simulink model "project2_sim"  (R2022b)
settings: Solver=VariableStepAuto  StartTime=0.0  StopTime=10.0  RelTol=1e-3
values from neighbouring files (symbols this model uses):
  A = [ ... (first row only)    [project2.m]    (also in project2_p1.m = A-B*K_reg; project2_p2.m = A-B*K_reg)
  Ad = [ ... (first row only)    [project2.m]    (also in project2_p2.m; set_topology.m)
  B = [ ... (first row only)    [project2.m]    (also in project2_p1.m; project2_p2.m)
  c = (0.5/min(real(eigs)))+ 0.5    [project2_p1.m]    (also in project2_p2.m = (0.5/min(real(eigs))) + 0.5)
  C = [708.27 0]    [project2.m]    (also in project2_p1.m; project2_p2.m)
  F = Pf*C'/R    [project2_p1.m]
  G = [ ... (first row only)    [project2.m]    (also in project2_p2.m = eye(6); set_topology.m = diag([1 0 0 0 0 1]))
  K = R\B'*P    [project2_p1.m]    (also in project2_p2.m = inv(R)*B'*P)
  K_reg = acker(A,B, [0 0])    [project2_p1.m]    (also in project2_p2.m)
  Lu_obs = (place(A', C', [-20, -10]))'    [project2_p1.m]
  xhat0 = [0 0]'    [project2_p1.m]    (also in project2_p2.m)
settings Model: Creator=simonecarena  LastModifiedBy=Enf
settings DebuggingCC: AlgebraicLoopMsg=none

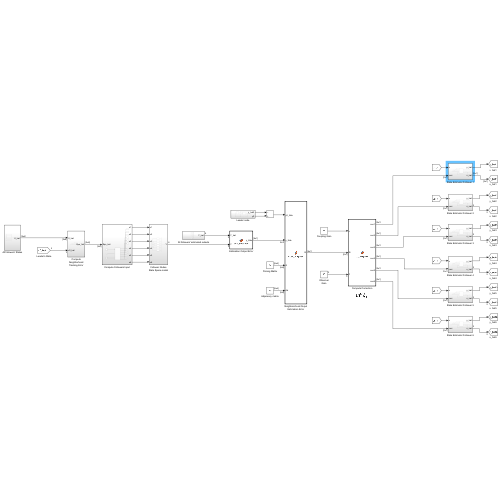
[thumbnail: Simulink's stored preview of the top-level diagram]
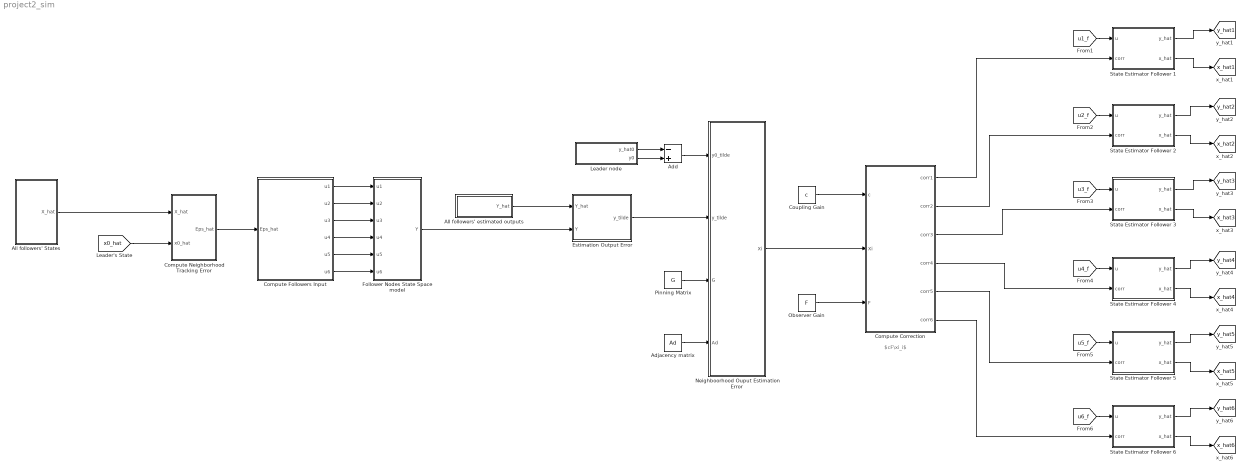
== system project2_sim ==
  note: $cF\xi_i$
  Add : Sum  Inputs=-+
  Adjacency matrix : Constant  Value=Ad
  All followers' States : Subsystem
  All followers' estimated outputs : Subsystem
  Compute Neighborhood Tracking Error : Subsystem
  Compute Correction : MATLAB Function  TreatAsAtomicUnit=on
  Compute Followers Input : Subsystem
  Coupling Gain : Constant  Value=c
  Estimation Output Error : MATLAB Function  TreatAsAtomicUnit=on
  Follower Nodes State Space model : Subsystem
  Leader node : Subsystem
  Neighboorhood Ouput Estimation Error : MATLAB Function  TreatAsAtomicUnit=on
  Observer Gain : Constant  Value=F
  Pinning Matrix : Constant  Value=G
  State Estimator Follower 1 : Subsystem
  State Estimator Follower 2 : Subsystem
  State Estimator Follower 3 : Subsystem
  State Estimator Follower 4 : Subsystem
  State Estimator Follower 5 : Subsystem
  State Estimator Follower 6 : Subsystem
  tag scope: x_hat1=global, x_hat2=global, x_hat3=global, x_hat4=global, x_hat5=global, x_hat6=global, y_hat1=global, y_hat2=global, y_hat3=global, y_hat4=global, y_hat5=global, y_hat6=global
  wires:
  Estimation Output Error/1(y_tilde) -> Neighboorhood Ouput Estimation Error/2(y_tilde)
  Adjacency matrix/1 -> Neighboorhood Ouput Estimation Error/4(Ad)
  Pinning Matrix/1 -> Neighboorhood Ouput Estimation Error/3(G)
  Add/1 -> Neighboorhood Ouput Estimation Error/1(y0_tilde)
  Neighboorhood Ouput Estimation Error/1(Xi) -> Compute Correction/2(Xi)
  Compute Correction/1(corr1) -> State Estimator Follower 1/2(corr)
  Compute Correction/2(corr2) -> State Estimator Follower 2/2(corr)
  Compute Correction/3(corr3) -> State Estimator Follower 3/2(corr)
  Compute Correction/4(corr4) -> State Estimator Follower 4/2(corr)
  Compute Correction/5(corr5) -> State Estimator Follower 5/2(corr)
  Compute Correction/6(corr6) -> State Estimator Follower 6/2(corr)
  State Estimator Follower 1/1(y_hat) -> [y_hat1]
  State Estimator Follower 3/1(y_hat) -> [y_hat3]
  State Estimator Follower 6/1(y_hat) -> [y_hat6]
  State Estimator Follower 5/1(y_hat) -> [y_hat5]
  State Estimator Follower 4/1(y_hat) -> [y_hat4]
  State Estimator Follower 2/1(y_hat) -> [y_hat2]
  All followers' estimated outputs/1(Y_hat) -> Estimation Output Error/1(Y_hat)
  State Estimator Follower 1/2(x_hat) -> [x_hat1]
  State Estimator Follower 2/2(x_hat) -> [x_hat2]
  State Estimator Follower 3/2(x_hat) -> [x_hat3]
  State Estimator Follower 4/2(x_hat) -> [x_hat4]
  State Estimator Follower 5/2(x_hat) -> [x_hat5]
  State Estimator Follower 6/2(x_hat) -> [x_hat6]
  Leader node/1(y_hat0) -> Add/1
  Leader node/2(y0) -> Add/2
  Observer Gain/1 -> Compute Correction/3(F)
  Coupling Gain/1 -> Compute Correction/1(c)
  All followers' States/1(X_hat) -> Compute Neighborhood Tracking Error/1(X_hat)
  [x0_hat] -> Compute Neighborhood Tracking Error/2(x0_hat)
  Compute Neighborhood Tracking Error/1(Eps_hat) -> Compute Followers Input/1(Eps_hat)
  [u4_f] -> State Estimator Follower 4/1(u)
  [u6_f] -> State Estimator Follower 6/1(u)
  [u5_f] -> State Estimator Follower 5/1(u)
  [u3_f] -> State Estimator Follower 3/1(u)
  [u1_f] -> State Estimator Follower 1/1(u)
  [u2_f] -> State Estimator Follower 2/1(u)
  Compute Followers Input/1(u1) -> Follower Nodes State Space model/1(u1)
  Compute Followers Input/2(u2) -> Follower Nodes State Space model/2(u2)
  Compute Followers Input/3(u3) -> Follower Nodes State Space model/3(u3)
  Compute Followers Input/4(u4) -> Follower Nodes State Space model/4(u4)
  Compute Followers Input/5(u5) -> Follower Nodes State Space model/5(u5)
  Compute Followers Input/6(u6) -> Follower Nodes State Space model/6(u6)
  Follower Nodes State Space model/1(Y) -> Estimation Output Error/2(Y)

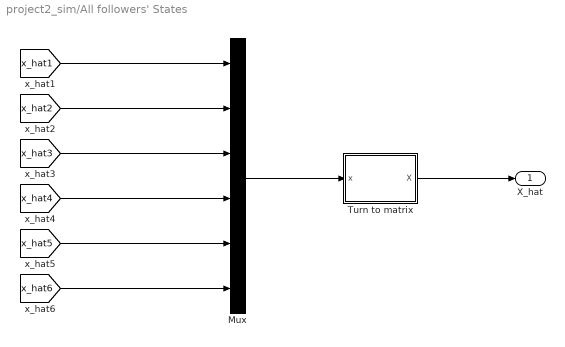
== system project2_sim/All followers' States ==
  Mux : Mux  Inputs=6
  Turn to matrix : MATLAB Function  TreatAsAtomicUnit=on
  X_hat : Outport
  wires:
  [x_hat1] -> Mux/1
  [x_hat2] -> Mux/2
  [x_hat3] -> Mux/3
  [x_hat4] -> Mux/4
  [x_hat5] -> Mux/5
  [x_hat6] -> Mux/6
  Mux/1 -> Turn to matrix/1(x)
  Turn to matrix/1(X) -> X_hat/1

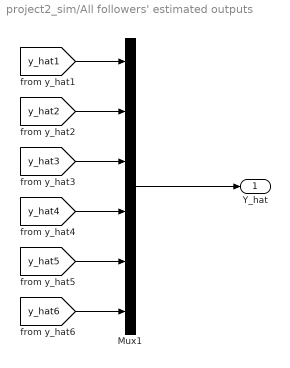
== system project2_sim/All followers' estimated outputs ==
  Mux1 : Mux  Inputs=6
  Y_hat : Outport
  wires:
  [y_hat6] -> Mux1/6
  [y_hat4] -> Mux1/4
  [y_hat1] -> Mux1/1
  [y_hat5] -> Mux1/5
  [y_hat3] -> Mux1/3
  Mux1/1 -> Y_hat/1
  [y_hat2] -> Mux1/2

== system project2_sim/Compute Neighborhood Tracking Error ==
  X_hat : Inport
  x0_hat : Inport  Port=2
  Constant1 : Constant  Value=G
  Neighborhood Tracking Error : MATLAB Function  TreatAsAtomicUnit=on
  adjacency matrix : Constant  Value=Ad
  Eps_hat : Outport
  wires:
  X_hat/1 -> Neighborhood Tracking Error/1(X_hat)
  x0_hat/1 -> Neighborhood Tracking Error/2(x0_hat)
  adjacency matrix/1 -> Neighborhood Tracking Error/3(Ad)
  Constant1/1 -> Neighborhood Tracking Error/4(G)
  Neighborhood Tracking Error/1(Eps) -> Eps_hat/1

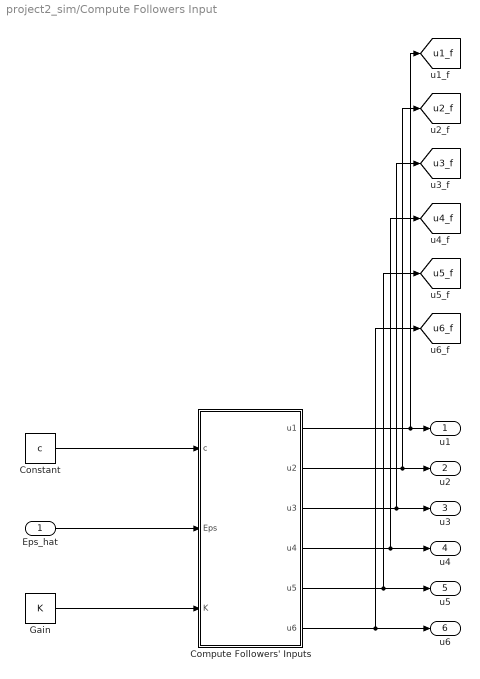
== system project2_sim/Compute Followers Input ==
  Eps_hat : Inport
  Compute Followers' Inputs : MATLAB Function  TreatAsAtomicUnit=on
  Constant : Constant  Value=c
  Gain : Constant  Value=K  VectorParams1D=off
  u1 : Outport
  u2 : Outport  Port=2
  u3 : Outport  Port=3
  u4 : Outport  Port=4
  u5 : Outport  Port=5
  u6 : Outport  Port=6
  tag scope: u1_f=global, u2_f=global, u3_f=global, u4_f=global, u5_f=global, u6_f=global
  wires:
  Eps_hat/1 -> Compute Followers' Inputs/2(Eps)
  Constant/1 -> Compute Followers' Inputs/1(c)
  Gain/1 -> Compute Followers' Inputs/3(K)
  Compute Followers' Inputs/1(u1) -> [u1_f], u1/1
  Compute Followers' Inputs/2(u2) -> u2/1, [u2_f]
  Compute Followers' Inputs/3(u3) -> u3/1, [u3_f]
  Compute Followers' Inputs/4(u4) -> u4/1, [u4_f]
  Compute Followers' Inputs/5(u5) -> u5/1, [u5_f]
  Compute Followers' Inputs/6(u6) -> [u6_f], u6/1

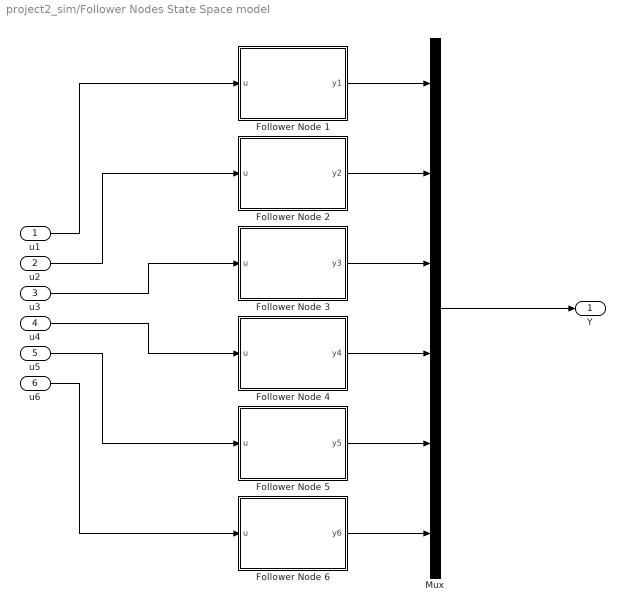
== system project2_sim/Follower Nodes State Space model ==
  u1 : Inport
  u2 : Inport  Port=2
  u3 : Inport  Port=3
  u4 : Inport  Port=4
  u5 : Inport  Port=5
  u6 : Inport  Port=6
  Follower Node 1 : Subsystem
  Follower Node 2 : Subsystem
  Follower Node 3 : Subsystem
  Follower Node 4 : Subsystem
  Follower Node 5 : Subsystem
  Follower Node 6 : Subsystem
  Mux : Mux  Inputs=6
  Y : Outport
  wires:
  Follower Node 4/1(y4) -> Mux/4
  Mux/1 -> Y/1
  u4/1 -> Follower Node 4/1(u)
  Follower Node 2/1(y2) -> Mux/2
  Follower Node 6/1(y6) -> Mux/6
  Follower Node 3/1(y3) -> Mux/3
  Follower Node 1/1(y1) -> Mux/1
  Follower Node 5/1(y5) -> Mux/5
  u5/1 -> Follower Node 5/1(u)
  u3/1 -> Follower Node 3/1(u)
  u2/1 -> Follower Node 2/1(u)
  u1/1 -> Follower Node 1/1(u)
  u6/1 -> Follower Node 6/1(u)

== system project2_sim/Leader node ==
  Gain : Gain  Gain=-K_reg  Multiplication=Matrix(K*u)
  Leader Node : Subsystem
  Leader Node Estimator : Subsystem
  y_hat0 : Outport
  y0 : Outport  Port=2
  wires:
  Leader Node Estimator/2(y_hat0) -> y_hat0/1
  Leader Node/1(y0) -> y0/1, Leader Node Estimator/1(y0)
  Gain/1 -> Leader Node/1(u), Leader Node Estimator/2(u)
  Leader Node Estimator/1(x_hat0) -> Gain/1

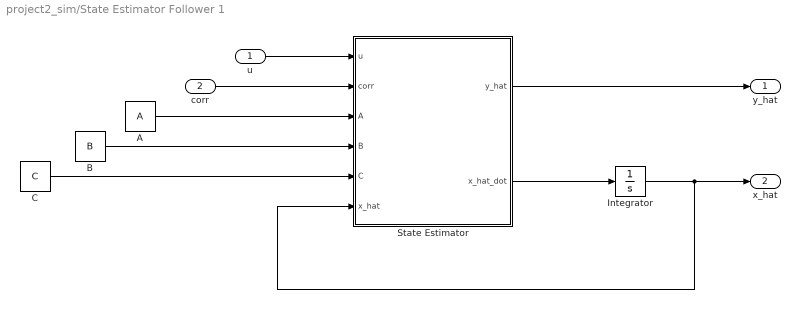
== system project2_sim/State Estimator Follower 1 ==
  u : Inport
  corr : Inport  Port=2
  A : Constant  Value=A
  B : Constant  Value=B  VectorParams1D=off
  C : Constant  Value=C  VectorParams1D=off
  Integrator : Integrator  InitialCondition=xhat0
  State Estimator : MATLAB Function  TreatAsAtomicUnit=on
  y_hat : Outport
  x_hat : Outport  Port=2
  wires:
  State Estimator/1(y_hat) -> y_hat/1
  u/1 -> State Estimator/1(u)
  corr/1 -> State Estimator/2(corr)
  State Estimator/2(x_hat_dot) -> Integrator/1
  Integrator/1 -> State Estimator/6(x_hat), x_hat/1
  A/1 -> State Estimator/3(A)
  B/1 -> State Estimator/4(B)
  C/1 -> State Estimator/5(C)

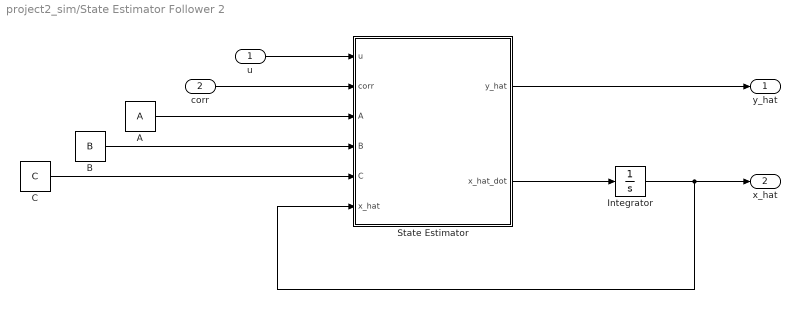
== system project2_sim/State Estimator Follower 2 ==
  u : Inport
  corr : Inport  Port=2
  A : Constant  Value=A
  B : Constant  Value=B  VectorParams1D=off
  C : Constant  Value=C  VectorParams1D=off
  Integrator : Integrator  InitialCondition=xhat0
  State Estimator : MATLAB Function  TreatAsAtomicUnit=on
  y_hat : Outport
  x_hat : Outport  Port=2
  wires:
  C/1 -> State Estimator/5(C)
  B/1 -> State Estimator/4(B)
  A/1 -> State Estimator/3(A)
  Integrator/1 -> x_hat/1, State Estimator/6(x_hat)
  State Estimator/2(x_hat_dot) -> Integrator/1
  corr/1 -> State Estimator/2(corr)
  u/1 -> State Estimator/1(u)
  State Estimator/1(y_hat) -> y_hat/1

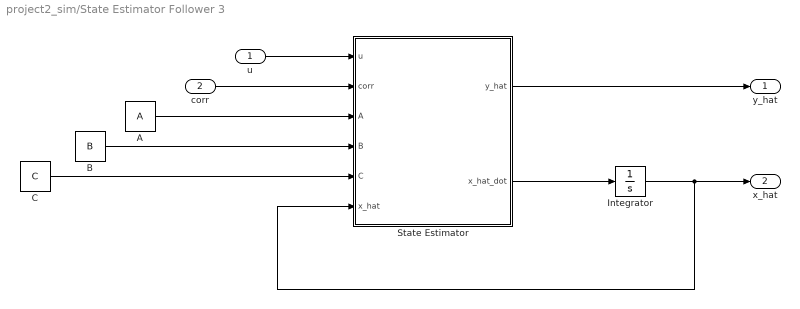
== system project2_sim/State Estimator Follower 3 ==
  u : Inport
  corr : Inport  Port=2
  A : Constant  Value=A
  B : Constant  Value=B  VectorParams1D=off
  C : Constant  Value=C  VectorParams1D=off
  Integrator : Integrator  InitialCondition=xhat0
  State Estimator : MATLAB Function  TreatAsAtomicUnit=on
  y_hat : Outport
  x_hat : Outport  Port=2
  wires:
  State Estimator/1(y_hat) -> y_hat/1
  u/1 -> State Estimator/1(u)
  corr/1 -> State Estimator/2(corr)
  State Estimator/2(x_hat_dot) -> Integrator/1
  Integrator/1 -> State Estimator/6(x_hat), x_hat/1
  A/1 -> State Estimator/3(A)
  B/1 -> State Estimator/4(B)
  C/1 -> State Estimator/5(C)

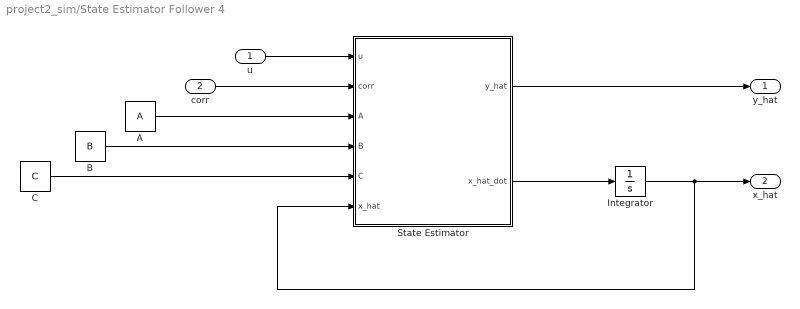
== system project2_sim/State Estimator Follower 4 ==
  u : Inport
  corr : Inport  Port=2
  A : Constant  Value=A
  B : Constant  Value=B  VectorParams1D=off
  C : Constant  Value=C  VectorParams1D=off
  Integrator : Integrator  InitialCondition=xhat0
  State Estimator : MATLAB Function  TreatAsAtomicUnit=on
  y_hat : Outport
  x_hat : Outport  Port=2
  wires:
  C/1 -> State Estimator/5(C)
  B/1 -> State Estimator/4(B)
  A/1 -> State Estimator/3(A)
  Integrator/1 -> x_hat/1, State Estimator/6(x_hat)
  State Estimator/2(x_hat_dot) -> Integrator/1
  corr/1 -> State Estimator/2(corr)
  u/1 -> State Estimator/1(u)
  State Estimator/1(y_hat) -> y_hat/1

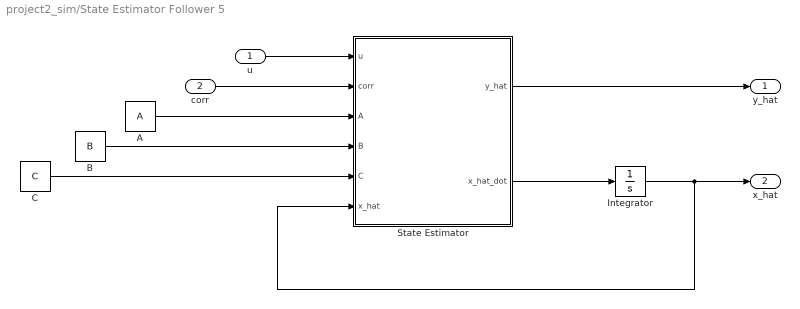
== system project2_sim/State Estimator Follower 5 ==
  u : Inport
  corr : Inport  Port=2
  A : Constant  Value=A
  B : Constant  Value=B  VectorParams1D=off
  C : Constant  Value=C  VectorParams1D=off
  Integrator : Integrator  InitialCondition=xhat0
  State Estimator : MATLAB Function  TreatAsAtomicUnit=on
  y_hat : Outport
  x_hat : Outport  Port=2
  wires:
  State Estimator/1(y_hat) -> y_hat/1
  u/1 -> State Estimator/1(u)
  corr/1 -> State Estimator/2(corr)
  State Estimator/2(x_hat_dot) -> Integrator/1
  Integrator/1 -> State Estimator/6(x_hat), x_hat/1
  A/1 -> State Estimator/3(A)
  B/1 -> State Estimator/4(B)
  C/1 -> State Estimator/5(C)

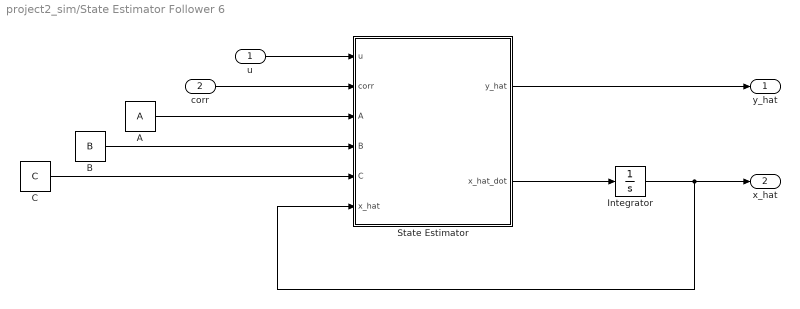
== system project2_sim/State Estimator Follower 6 ==
  u : Inport
  corr : Inport  Port=2
  A : Constant  Value=A
  B : Constant  Value=B  VectorParams1D=off
  C : Constant  Value=C  VectorParams1D=off
  Integrator : Integrator  InitialCondition=xhat0
  State Estimator : MATLAB Function  TreatAsAtomicUnit=on
  y_hat : Outport
  x_hat : Outport  Port=2
  wires:
  C/1 -> State Estimator/5(C)
  B/1 -> State Estimator/4(B)
  A/1 -> State Estimator/3(A)
  Integrator/1 -> x_hat/1, State Estimator/6(x_hat)
  State Estimator/2(x_hat_dot) -> Integrator/1
  corr/1 -> State Estimator/2(corr)
  u/1 -> State Estimator/1(u)
  State Estimator/1(y_hat) -> y_hat/1

== system project2_sim/Follower Nodes State Space model/Follower Node 1 ==
  u : Inport
  State-Space : StateSpace  A=A  B=B  C=C  D=0  InitialCondition=0
  y1 : Outport
  wires:
  u/1 -> State-Space/1
  State-Space/1 -> y1/1

== system project2_sim/Follower Nodes State Space model/Follower Node 2 ==
  u : Inport
  State-Space : StateSpace  A=A  B=B  C=C  D=0  InitialCondition=0
  y2 : Outport
  wires:
  u/1 -> State-Space/1
  State-Space/1 -> y2/1

== system project2_sim/Follower Nodes State Space model/Follower Node 3 ==
  u : Inport
  State-Space : StateSpace  A=A  B=B  C=C  D=0  InitialCondition=0
  y3 : Outport
  wires:
  u/1 -> State-Space/1
  State-Space/1 -> y3/1

== system project2_sim/Follower Nodes State Space model/Follower Node 4 ==
  u : Inport
  State-Space : StateSpace  A=A  B=B  C=C  D=0  InitialCondition=0
  y4 : Outport
  wires:
  u/1 -> State-Space/1
  State-Space/1 -> y4/1

== system project2_sim/Follower Nodes State Space model/Follower Node 5 ==
  u : Inport
  State-Space : StateSpace  A=A  B=B  C=C  D=0  InitialCondition=0
  y5 : Outport
  wires:
  State-Space/1 -> y5/1
  u/1 -> State-Space/1

== system project2_sim/Follower Nodes State Space model/Follower Node 6 ==
  u : Inport
  State-Space : StateSpace  A=A  B=B  C=C  D=0  InitialCondition=0
  y6 : Outport
  wires:
  u/1 -> State-Space/1
  State-Space/1 -> y6/1

== system project2_sim/Leader node/Leader Node ==
  u : Inport
  State-Space : StateSpace  A=A  B=B  C=C  D=0  InitialCondition=0
  y0 : Outport
  wires:
  u/1 -> State-Space/1
  State-Space/1 -> y0/1

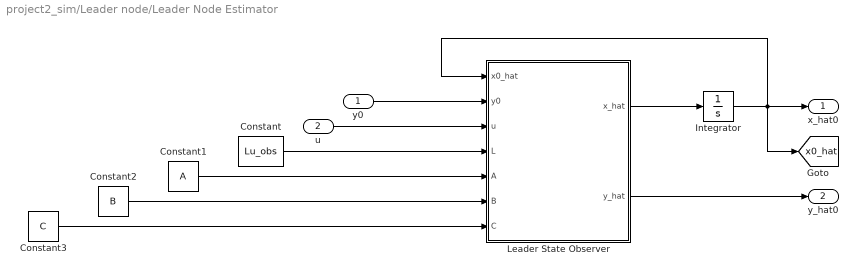
== system project2_sim/Leader node/Leader Node Estimator ==
  y0 : Inport
  u : Inport  Port=2
  Constant : Constant  Value=Lu_obs  VectorParams1D=off
  Constant1 : Constant  Value=A
  Constant2 : Constant  Value=B  VectorParams1D=off
  Constant3 : Constant  Value=C  VectorParams1D=off
  Integrator : Integrator  InitialCondition=[0; 0]
  Leader State Observer : MATLAB Function  TreatAsAtomicUnit=on
  x_hat0 : Outport
  y_hat0 : Outport  Port=2
  tag scope: x0_hat=global
  wires:
  u/1 -> Leader State Observer/3(u)
  y0/1 -> Leader State Observer/2(y0)
  Leader State Observer/2(y_hat) -> y_hat0/1
  Constant/1 -> Leader State Observer/4(L)
  Leader State Observer/1(x_hat) -> Integrator/1
  Integrator/1 -> [x0_hat], Leader State Observer/1(x0_hat), x_hat0/1
  Constant1/1 -> Leader State Observer/5(A)
  Constant2/1 -> Leader State Observer/6(B)
  Constant3/1 -> Leader State Observer/7(C)

== matlab function project2_sim/State Estimator Follower 6/State Estimator ==
  data: y_hat output; u input; x_hat_dot output; corr input; A input; B input; C input; x_hat input
function [y_hat, x_hat_dot] = state_estimator_wrapper(u, corr, A, B, C, x_hat)
    [y_hat, x_hat_dot] = state_estimator(u, corr, A, B, C, x_hat);
return

== matlab function project2_sim/Leader node/Leader Node Estimator/Leader State Observer ==
  data: x0_hat input; y0 input; u input; x_hat output; y_hat output; L input; A input; B input; C input
function [x_hat, y_hat] = leader_state_obs_wrapper(x0_hat, y0, u, L, A, B, C)
    [x_hat, y_hat] = leader_state_obs(x0_hat, y0, u, L, A, B, C);
return

== matlab function project2_sim/All followers' States/Turn to matrix ==
  data: x input; X output
function X = turnToMatrix(x)

    X = reshape(x,2,6);

== matlab function project2_sim/Compute Neighborhood Tracking Error/Neighborhood Tracking Error ==
  data: X_hat input; Eps output; x0_hat input; Ad input; G input
function Eps = nte_wrapper(X_hat, x0_hat, Ad, G)

    Eps = zeros(2,6);

    for i=1:6
       Eps(:,i) = nte(Ad,G,x0_hat,X_hat,i);
    end

== matlab function project2_sim/Neighboorhood Ouput Estimation Error ==
  data: y0_tilde input; Xi output; y_tilde input; G input; Ad input
function Xi = noer_wrapper(y0_tilde, y_tilde, G, Ad)

    Xi = zeros(6, 1);

    for i=1:6
        Xi(:, i) = noer(Ad,G,y0_tilde,y_tilde,i);
    end

== matlab function project2_sim/Compute Followers Input/Compute Followers' Inputs ==
  data: c input; Eps input; u1 output; u2 output; u3 output; u4 output; u5 output; u6 output; K input
function [u1, u2, u3, u4, u5, u6] = ui(c,Eps,K)

    u1 = 0;
    u2 = 0;
    u3 = 0;
    u4 = 0;
    u5 = 0;
    u6 = 0;

    u1 = c*K*Eps(:, 1);
    u2 = c*K*Eps(:, 2);
    u3 = c*K*Eps(:, 3);
    u4 = c*K*Eps(:, 4);
    u5 = c*K*Eps(:, 5);
    u6 = c*K*Eps(:, 6);

== matlab function project2_sim/Estimation Output Error ==
  data: Y_hat input; y_tilde output; Y input
function y_tilde = eoe_wrapper(Y_hat, Y)
   y_tilde = eoe(Y_hat, Y);
end

== matlab function project2_sim/Compute Correction ==
  data: c input; Xi input; corr1 output size=[2 1]; F input; corr2 output; corr3 output; corr4 output; corr5 output; corr6 output
function [corr1, corr2, corr3, corr4, corr5, corr6]  = cc_wrapper(c, Xi, F)
    corr1 = zeros(2, 1);
    corr2 = zeros(2, 1);
    corr3 = zeros(2, 1);
    corr4 = zeros(2, 1);
    corr5 = zeros(2, 1);
    corr6 = zeros(2, 1);

    [corr1,corr2,corr3,corr4,corr5,corr6] = compute_correction(c, Xi, F);
end

== matlab function project2_sim/State Estimator Follower 1/State Estimator ==
  data: y_hat output; u input; x_hat_dot output; corr input; A input; B input; C input; x_hat input
function [y_hat, x_hat_dot] = state_estimator_wrapper(u, corr, A, B, C, x_hat)
    [y_hat, x_hat_dot] = state_estimator(u, corr, A, B, C, x_hat);
return

== matlab function project2_sim/State Estimator Follower 2/State Estimator ==
  data: y_hat output; u input; x_hat_dot output; corr input; A input; B input; C input; x_hat input
function [y_hat, x_hat_dot] = state_estimator_wrapper(u, corr, A, B, C, x_hat)
    [y_hat, x_hat_dot] = state_estimator(u, corr, A, B, C, x_hat);
return

== matlab function project2_sim/State Estimator Follower 3/State Estimator ==
  data: y_hat output; u input; x_hat_dot output; corr input; A input; B input; C input; x_hat input
function [y_hat, x_hat_dot] = state_estimator_wrapper(u, corr, A, B, C, x_hat)
    [y_hat, x_hat_dot] = state_estimator(u, corr, A, B, C, x_hat);
return

== matlab function project2_sim/State Estimator Follower 4/State Estimator ==
  data: y_hat output; u input; x_hat_dot output; corr input; A input; B input; C input; x_hat input
function [y_hat, x_hat_dot] = state_estimator_wrapper(u, corr, A, B, C, x_hat)
    [y_hat, x_hat_dot] = state_estimator(u, corr, A, B, C, x_hat);
return

== matlab function project2_sim/State Estimator Follower 5/State Estimator ==
  data: y_hat output; u input; x_hat_dot output; corr input; A input; B input; C input; x_hat input
function [y_hat, x_hat_dot] = state_estimator_wrapper(u, corr, A, B, C, x_hat)
    [y_hat, x_hat_dot] = state_estimator(u, corr, A, B, C, x_hat);
return
